simulink model "i_control"  (R2022a)
settings: Solver=ode4  StartTime=0.0  StopTime=10.0  FixedStep=0.01  RelTol=1e-3
values from neighbouring files (symbols this model uses):
  den = [1  N]    [PD_only.m]    (also in PI_only.m = [1 0])
  Ki = K(i)    [PI_only.m]    (also in Pi_control_script.m; i_control_script.m)
  num = [Kp+Kd*N  Kp*N]    [PD_control_script.m]    (also in PD_only.m = [Kp+Kd*N N]; PI_only.m = [Kp  Ki]; Pi_control_script.m = [Kp Ki]; i_control_script.m = Ki)
settings Model: Creator=김응태  LastModifiedBy=ADMIN

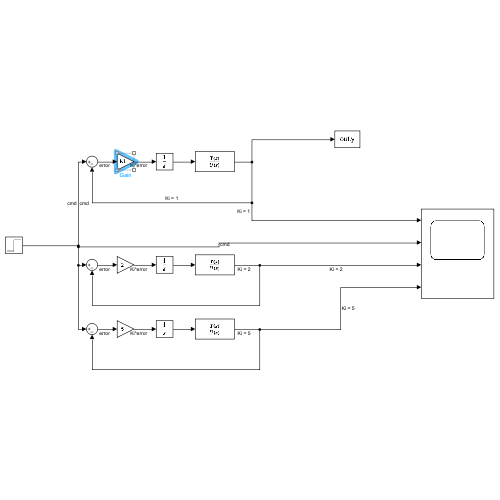
[thumbnail: Simulink's stored preview of the top-level diagram]
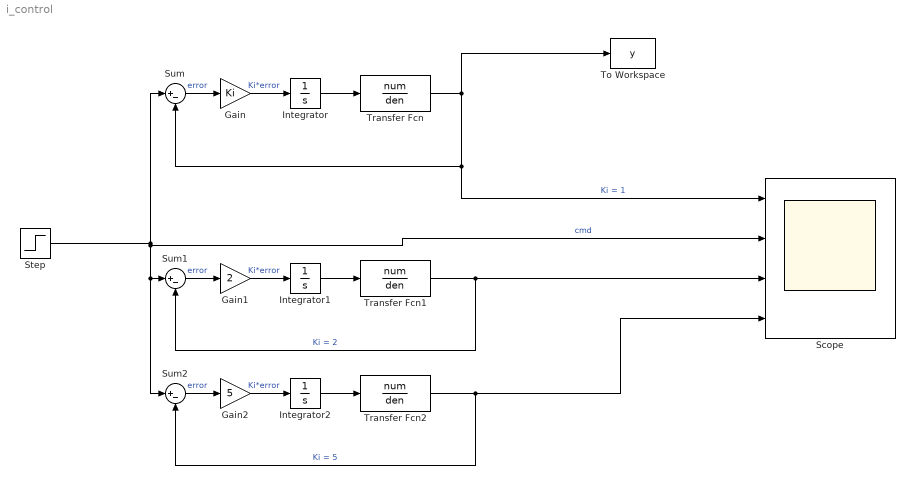
== system i_control ==
  Gain : Gain  Gain=Ki
  Gain1 : Gain  Gain=2
  Gain2 : Gain  Gain=5
  Integrator : Integrator
  Integrator1 : Integrator
  Integrator2 : Integrator
  Scope : Scope  NumInputPorts=4
  Step : Step  Time=2  SampleTime=0
  Sum : Sum  Inputs=|+-
  Sum1 : Sum  Inputs=|+-
  Sum2 : Sum  Inputs=|+-
  To Workspace : ToWorkspace  VariableName=y  SaveFormat=Timeseries  SampleTime=-1
  Transfer Fcn : TransferFcn  Numerator=num  Denominator=den
  Transfer Fcn1 : TransferFcn  Numerator=num  Denominator=den
  Transfer Fcn2 : TransferFcn  Numerator=num  Denominator=den
  wires:
  Gain/1 -> Integrator/1  "Ki*error"
  Sum/1 -> Gain/1  "error"
  Step/1 -> Sum2/1, Sum1/1, Scope/2, Sum/1  "cmd"
  Transfer Fcn/1 -> Scope/1, Sum/2, To Workspace/1  "Ki = 1"
  Integrator/1 -> Transfer Fcn/1
  Sum1/1 -> Gain1/1  "error"
  Gain1/1 -> Integrator1/1  "Ki*error"
  Integrator1/1 -> Transfer Fcn1/1
  Transfer Fcn1/1 -> Sum1/2, Scope/3  "Ki = 2"
  Sum2/1 -> Gain2/1  "error"
  Transfer Fcn2/1 -> Sum2/2, Scope/4  "Ki = 5"
  Integrator2/1 -> Transfer Fcn2/1
  Gain2/1 -> Integrator2/1  "Ki*error"
